simulink library "INT_SmkLim_InjMassLim"  (R2016b)
settings: Solver=VariableStepAuto  StartTime=0.0  StopTime=10.0  RelTol=1e-3
settings Model: Creator=xuxingpei  LastModifiedBy=xuxingpei

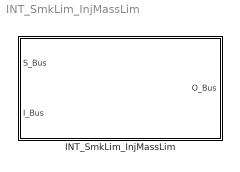
== system INT_SmkLim_InjMassLim ==
  INT_SmkLim_InjMassLim : Subsystem

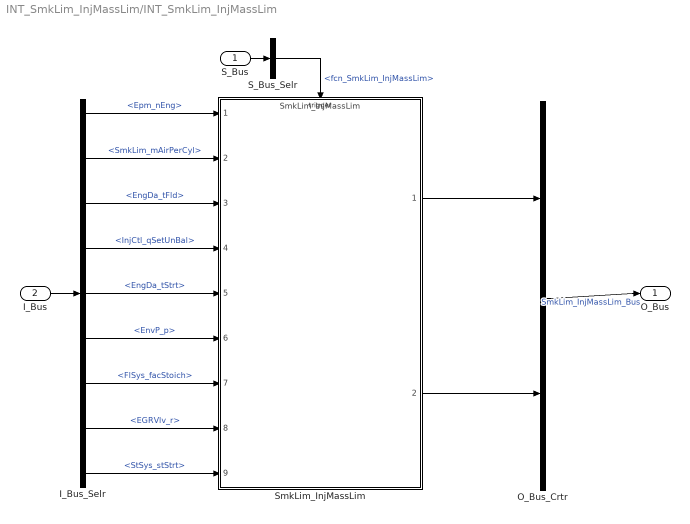
== system INT_SmkLim_InjMassLim/INT_SmkLim_InjMassLim ==
  S_Bus : Inport
  I_Bus : Inport  Port=2
  I_Bus_Selr : BusSelector  OutputSignals=Epm_nEng,SmkLim_mAirPerCyl,EngDa_tFld,InjCtl_qSetUnBal,EngDa_tStrt,EnvP_p,FlSys_facStoich,EGRVlv_r,StSys_stStrt
  O_Bus_Crtr : BusCreator  Inputs=2
  S_Bus_Selr : BusSelector  OutputSignals=fcn_SmkLim_InjMassLim
  SmkLim_InjMassLim : ModelReference  ModelNameDialog=SmkLim_InjMassLim  SimulationMode=Normal  ModelReferenceVersion=1.51  TriggerPortName=function  TriggerPortTriggerType=function-call  TriggerPortStatesWhenEnabling=held
  O_Bus : Outport
  wires:
  S_Bus_Selr/1 -> SmkLim_InjMassLim/Trigger  "<fcn_SmkLim_InjMassLim>"
  S_Bus/1 -> S_Bus_Selr/1
  I_Bus/1 -> I_Bus_Selr/1
  I_Bus_Selr/1 -> SmkLim_InjMassLim/1  "<Epm_nEng>"
  I_Bus_Selr/2 -> SmkLim_InjMassLim/2  "<SmkLim_mAirPerCyl>"
  I_Bus_Selr/3 -> SmkLim_InjMassLim/3  "<EngDa_tFld>"
  I_Bus_Selr/4 -> SmkLim_InjMassLim/4  "<InjCtl_qSetUnBal>"
  I_Bus_Selr/5 -> SmkLim_InjMassLim/5  "<EngDa_tStrt>"
  I_Bus_Selr/6 -> SmkLim_InjMassLim/6  "<EnvP_p>"
  I_Bus_Selr/7 -> SmkLim_InjMassLim/7  "<FlSys_facStoich>"
  I_Bus_Selr/8 -> SmkLim_InjMassLim/8  "<EGRVlv_r>"
  I_Bus_Selr/9 -> SmkLim_InjMassLim/9  "<StSys_stStrt>"
  O_Bus_Crtr/1 -> O_Bus/1  "SmkLim_InjMassLim_Bus"
  SmkLim_InjMassLim/1 -> O_Bus_Crtr/1
  SmkLim_InjMassLim/2 -> O_Bus_Crtr/2
